simulink model "qdr_5_5"  (Simulink 7.9)
settings: Solver=ode45  StartTime=0.0  StopTime=10.0  RelTol=1e-3
libraries: xbsIndex_r4 x44, xps_library x2, casper_library_delays x2, casper_library_misc x1
settings Model: Creator=tfiliba  LastModifiedBy=tfiliba

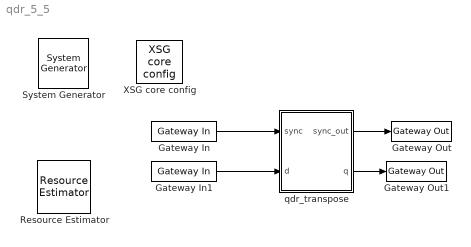
== system qdr_5_5 ==
  " System Generator" : xbsIndex_r4/ System Generator  Tag=genX  xilinxfamily=virtex5  part=xc5vsx95t  speed=-1  package=ff1136  synthesis_tool=XST  clock_wrapper=Clock Enables  directory=./netlist  proj_type=Project Navigator  Synth_file=XST Defaults  Impl_file=ISE Defaults  testbench=off  simulink_period=1  sysclk_period=10  dcm_input_clock_period=10  incr_netlist=off  trim_vbits=Everywhere in SubSystem  dbl_ovrd=According to Block Masks  core_generation=According to Block Masks  run_coregen=off  deprecated_control=off  eval_field=0  block_type=sysgen
  Gateway In : xbsIndex_r4/Gateway In  gui_display_data_type=Boolean  arith_type=Boolean  n_bits=16  bin_pt=14  preci_type=Single  exp_width=8  frac_width=24  quantization="Round  (unbiased: +/- Inf)"  overflow=Saturate  period=1  dbl_ovrd=off  timing_constraint=None  locs_specified=off  LOCs={}  UseAsADC=off  ADCChannel='1'  inherit_from_input=off  hdl_port=on  block_type=gatewayin
      settings: xl_area=[0 0 0 0 1 0 0]
  Gateway In1 : xbsIndex_r4/Gateway In  gui_display_data_type=Fixed-point  arith_type=Unsigned  n_bits=16  bin_pt=0  preci_type=Single  exp_width=8  frac_width=24  quantization="Round  (unbiased: +/- Inf)"  overflow=Saturate  period=1  dbl_ovrd=off  timing_constraint=None  locs_specified=off  LOCs={}  UseAsADC=off  ADCChannel='1'  inherit_from_input=off  hdl_port=on  block_type=gatewayin
      settings: xl_area=[0 0 0 0 16 0 0]
  Gateway Out : xbsIndex_r4/Gateway Out  inherit_from_input=off  hdl_port=on  timing_constraint=None  locs_specified=off  LOCs={}  UseAsDAC=off  DACChannel='1'  block_type=gatewayout
      settings: xl_area=[0 0 0 0 1 0 0]
  Gateway Out1 : xbsIndex_r4/Gateway Out  inherit_from_input=off  hdl_port=on  timing_constraint=None  locs_specified=off  LOCs={}  UseAsDAC=off  DACChannel='1'  block_type=gatewayout
      settings: xl_area=[0 0 0 0 36 0 0]
  Resource Estimator : xbsIndex_r4/Resource Estimator  Tag=resEstTag  Slices=0  FFs=0  BRAMs=0  LUTs=0  IOBs=0  EBMs=0  TBUFs=0  xl_use_estimator_area=off  est_options=Estimate  xl_estimator_area=[167 227 2 301 167 0 0]  block_type=resource_estimator
      settings: AttributesFormatString=Resource\nEstimator
  XSG core config : xps_library/XSG core config  Tag=xps:xsg  hw_sys=ROACH:sx95t  clk_src=arb_clk  ROACH_clk_src=arb_clk  ROACH2_clk_src=adc0_clk  clk_rate=200  sample_period=1  synthesis_tool=XST
  qdr_transpose : Subsystem  AncestorBlock=casper_library_reorder/qdr_transpose  mask{idepth=5, odepth=5, which_qdr=qdr1}
      mask prompts: idepth "Input blocksize (2^n)"; odepth "Output blocksize (2^n)"; which_qdr "QDR Chip"
      mask init:
      | new_map = tostring([[0:2^odepth-1]*2 [0:2^odepth-1]*2 + 1]);
      | set_param([gcb, '/reorder'], 'map', new_map);
      | set_param([gcb, '/qdr'], 'which_qdr', which_qdr);
      mask StyleString: edit,edit,popup(qdr0|qdr1)
  wires:
  Gateway In/1 -> qdr_transpose/1(sync)
  Gateway In1/1 -> qdr_transpose/2(d)
  qdr_transpose/1(sync_out) -> Gateway Out/1
  qdr_transpose/2(q) -> Gateway Out1/1

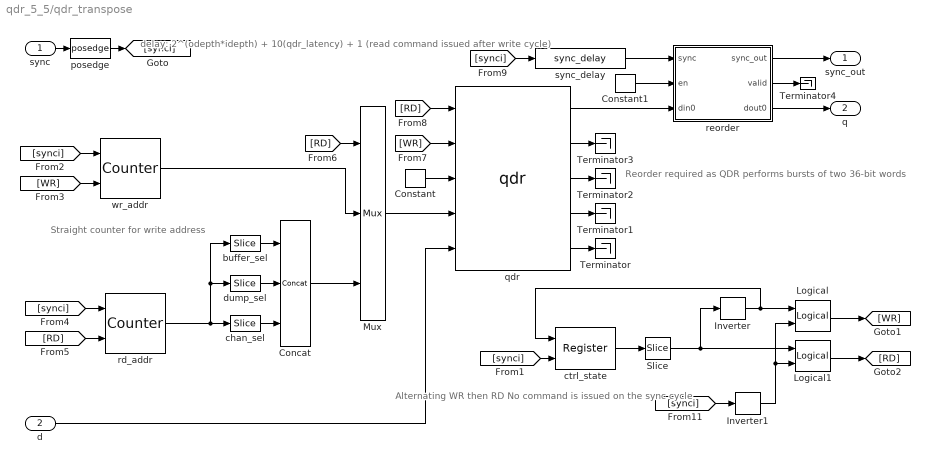
== system qdr_5_5/qdr_transpose ==
  note: delay: 2^(odepth*idepth) + 10(qdr_latency) + 1
      | (read command issued after write cycle)
  note: Reorder required as QDR performs
      | bursts of two 36-bit words
  note: Alternating WR then RD
      | No command is issued
      | on the sync cycle
  note: Straight counter for
      | write address
  sync : Inport
  d : Inport  Port=2
  Concat : xbsIndex_r4/Concat  num_inputs=3  dbl_ovrd=off  block_type=concat
      settings: block_version=10.1.3
  Constant : xbsIndex_r4/Constant  const=15  gui_display_data_type=Fixed-point  arith_type=Unsigned  n_bits=4  bin_pt=0  preci_type=Single  exp_width=8  frac_width=24  explicit_period=on  period=1  equ=P=C  opselect=C  inp2=PCIN>>17  opr=+  inp1=P  carry=CIN  dbl_ovrd=off  block_type=constant
  Constant1 : xbsIndex_r4/Constant  const=1  gui_display_data_type=Fixed-point  arith_type=Boolean  n_bits=4  bin_pt=0  preci_type=Single  exp_width=8  frac_width=24  explicit_period=on  period=1  equ=P=C  opselect=C  inp2=PCIN>>17  opr=+  inp1=P  carry=CIN  dbl_ovrd=off  block_type=constant
  Inverter : xbsIndex_r4/Inverter  en=off  latency=0  dbl_ovrd=off  block_type=inv
      settings: xl_area=[0 0 0 0 0 0 0]
  Inverter1 : xbsIndex_r4/Inverter  en=off  latency=0  dbl_ovrd=off  block_type=inv
      settings: xl_area=[0 0 0 0 0 0 0]
  Logical : xbsIndex_r4/Logical  logical_function=AND  inputs=2  en=off  latency=0  precision=Full  arith_type=Unsigned  n_bits=16  bin_pt=0  align_bp=on  dbl_ovrd=off  block_type=logical
      settings: xl_area=[1 0 0 1 0 0 0]
  Logical1 : xbsIndex_r4/Logical  logical_function=AND  inputs=2  en=off  latency=0  precision=Full  arith_type=Unsigned  n_bits=16  bin_pt=0  align_bp=on  dbl_ovrd=off  block_type=logical
      settings: xl_area=[1 0 0 1 0 0 0]
  Mux : xbsIndex_r4/Mux  inputs=2  en=off  latency=0  precision=Full  arith_type=Unsigned  n_bits=16  bin_pt=14  quantization=Truncate  overflow=Wrap  dbl_ovrd=off  block_type=mux
      settings: xl_area=[5 0 0 10 0 0 0]
  Slice : xbsIndex_r4/Slice  nbits=1  boolean_output=on  mode=Lower Bit Location + Width  bit1=0  base1=MSB of Input  bit0=0  base0=LSB of Input  dbl_ovrd=off  block_type=slice
      settings: infoedit="Extracts a given range of bits from each input sample and presents it at the output.  The output type is ordinarily unsigned with binary point at zero, but can be Boolean when the slice is one bit wide.<P><P>Hardware notes: In hardware this block costs nothing."  block_version=10.1.3
  Terminator{,1..4} (5 alike) : Terminator
  buffer_sel : xbsIndex_r4/Slice  nbits=1  boolean_output=off  mode=Upper Bit Location + Width  bit1=0  base1=MSB of Input  bit0=0  base0=LSB of Input  dbl_ovrd=off  block_type=slice
      settings: infoedit="Extracts a given range of bits from each input sample and presents it at the output.  The output type is ordinarily unsigned with binary point at zero, but can be Boolean when the slice is one bit wide.<P><P>Hardware notes: In hardware this block costs nothing."  block_version=10.1.3
  chan_sel : xbsIndex_r4/Slice  nbits=idepth - 1  boolean_output=off  mode=Lower Bit Location + Width  bit1=9-1  base1=MSB of Input  bit0=odepth  base0=LSB of Input  dbl_ovrd=off  block_type=slice
      settings: infoedit="Extracts a given range of bits from each input sample and presents it at the output.  The output type is ordinarily unsigned with binary point at zero, but can be Boolean when the slice is one bit wide.<P><P>Hardware notes: In hardware this block costs nothing."  block_version=10.1.3
  ctrl_state : xbsIndex_r4/Register  init=0  rst=on  en=off  dbl_ovrd=off  block_type=register
      settings: xl_area=[1 1 0 0 0 0 0]
  dump_sel : xbsIndex_r4/Slice  nbits=odepth  boolean_output=off  mode=Lower Bit Location + Width  bit1=0  base1=MSB of Input  bit0=0  base0=LSB of Input  dbl_ovrd=off  block_type=slice
      settings: infoedit="Extracts a given range of bits from each input sample and presents it at the output.  The output type is ordinarily unsigned with binary point at zero, but can be Boolean when the slice is one bit wide.<P><P>Hardware notes: In hardware this block costs nothing."  block_version=10.1.3
  posedge : casper_library_misc/posedge  Tag=Rising Edge Detector
      link override Delay: xl_area=[1 1 0 0 0 0 0]
      link override Inverter: xl_area=[0 0 0 0 0 0 0]
      link override Logical: xl_area=[1 0 0 1 0 0 0]
  qdr : xps_library/qdr  Tag=xps:qdr  which_qdr=qdr1  qdr_awidth=odepth+idepth+1  use_sniffer=off
      link override convert_be: n_bits=4
      link override convert_data_in: n_bits=36
      link override convert_data_in1: n_bits=36
      link override extract_parity: bitexpr=b = {a[35],a[26],a[17],a[8],a[34:27],a[25:18],a[16:9],a[7:0]}  arith_type1=Unsigned  arith_type2=Unsigned  arith_type3=Unsigned  arith_type4=Unsigned
      link override insert_parity: bitexpr=b = {a[35],a[31:24],a[34],a[23:16],a[33],a[15:8],a[32],a[7:0]}  arith_type1=Unsigned  arith_type2=Unsigned  arith_type3=Unsigned  arith_type4=Unsigned
      link override qdr_12_15_qdr_transpose_qdr_data_out: n_bits=36
      link override qdr_5_5_qdr_transpose_qdr_data_out: n_bits=36
      link override qdr_latency: latency=10
      link override Delay1: xl_area=[1 1 0 0 0 0 0]
      link override Inverter2: xl_area=[0 0 0 0 0 0 0]
      link override Logical: xl_area=[1 0 0 1 0 0 0]
      link override Logical1: xl_area=[1 0 0 1 0 0 0]
      link override convert_ack: xl_area=[0 0 0 0 0 0 0]
      link override convert_address: xl_area=[0 0 0 0 0 0 0]
      link override convert_be: xl_area=[0 0 0 0 0 0 0]
      link override convert_cal_fail: xl_area=[0 0 0 0 0 0 0]
      link override convert_data_in: xl_area=[0 0 0 0 0 0 0]
      link override convert_data_in1: xl_area=[0 0 0 0 0 0 0]
      link override convert_rd_en: xl_area=[0 0 0 0 0 0 0]
      link override convert_ready: xl_area=[0 0 0 0 0 0 0]
      link override convert_wr_en: xl_area=[0 0 0 0 0 0 0]
      link override prev_rd: xl_area=[1 1 0 0 0 0 0]
      link override qdr_12_15_qdr_transpose_qdr_ack: xl_area=[0 0 0 0 1 0 0]
      link override qdr_12_15_qdr_transpose_qdr_address: xl_area=[0 0 0 0 32 0 0]
      link override qdr_12_15_qdr_transpose_qdr_be: xl_area=[0 0 0 0 4 0 0]
      link override qdr_12_15_qdr_transpose_qdr_cal_fail: xl_area=[0 0 0 0 1 0 0]
      link override qdr_12_15_qdr_transpose_qdr_data_in: xl_area=[0 0 0 0 36 0 0]
      link override qdr_12_15_qdr_transpose_qdr_data_out: xl_area=[0 0 0 0 36 0 0]
      link override qdr_12_15_qdr_transpose_qdr_phy_ready: xl_area=[0 0 0 0 1 0 0]
      link override qdr_12_15_qdr_transpose_qdr_rd_en: xl_area=[0 0 0 0 1 0 0]
      link override qdr_12_15_qdr_transpose_qdr_wr_en: xl_area=[0 0 0 0 1 0 0]
      link override qdr_5_5_qdr_transpose_qdr_ack: xl_area=[0 0 0 0 1 0 0]
      link override qdr_5_5_qdr_transpose_qdr_address: xl_area=[0 0 0 0 32 0 0]
      link override qdr_5_5_qdr_transpose_qdr_be: xl_area=[0 0 0 0 4 0 0]
      link override qdr_5_5_qdr_transpose_qdr_cal_fail: xl_area=[0 0 0 0 1 0 0]
      link override qdr_5_5_qdr_transpose_qdr_data_in: xl_area=[0 0 0 0 36 0 0]
      link override qdr_5_5_qdr_transpose_qdr_data_out: xl_area=[0 0 0 0 36 0 0]
      link override qdr_5_5_qdr_transpose_qdr_phy_ready: xl_area=[0 0 0 0 1 0 0]
      link override qdr_5_5_qdr_transpose_qdr_rd_en: xl_area=[0 0 0 0 1 0 0]
      link override qdr_5_5_qdr_transpose_qdr_wr_en: xl_area=[0 0 0 0 1 0 0]
      link override qdr_latency: xl_area=[1 1 0 1 0 0 0]
  rd_addr : xbsIndex_r4/Counter  cnt_type=Free Running  cnt_to=Inf  operation=Up  start_count=2^(odepth + idepth - 1)  cnt_by_val=1  arith_type=Unsigned  n_bits=(idepth + odepth + 1) - 1  bin_pt=0  load_pin=off  rst=on  en=on  explicit_period=on  period=1  dbl_ovrd=off  use_behavioral_HDL=off  implementation=Fabric  use_rpm=off  block_type=counter
      settings: xl_area=[6 10 0 10 0 0 0]
  reorder : Subsystem  AncestorBlock=casper_library_reorder/reorder  mask(reorder){map=[0                                      2                                      4                                      6                                      8                                     10                                     12                                     14                                     16                                     18                                     20                                     22                                     24                                     26                                     28                                     30                                     32                                     34                                     36                                     38                                     40                                     42                                     44                                     46                                     48                                     50                                     52                                     54                                     56                                     58                                     60                                     62                                      1                                      3                                      5                                      7                                      9                                     11                                     13                                     15                                     17                                     19                                     21                                     23                                     25                                     27                                     29                                     31                                     33                                     35                                     37                                     39                                     41                                     43                                     45                                     47                                     49                                     51                                     53                                     55                                     57                                     59                                     61                                     63], n_inputs=1, bram_latency=2, map_latency=3, double_buffer=0, bram_map=off}
      mask prompts: map "Output Order:"; n_inputs "Number of inputs"; bram_latency "BRAM Latency"; map_latency "Map Latency"; double_buffer "Double Buffer"; bram_map "Use BlockRAM for Map"
      mask init:
      | reorder_init(gcb, ...
      |     'map', map, ...
      |     'n_inputs', n_inputs, ...
      |     'bram_latency', bram_latency, ...
      |     'map_latency', map_latency, ...
      |     'double_buffer', double_buffer, ...
      |     'bram_map', bram_map);
      settings: AttributesFormatString=order=6
      mask Help: eval('xlWeb(''http://casper.berkeley.edu/wiki/Reorder'')')
  sync_delay : casper_library_delays/sync_delay  DelayLen=2^(idepth + odepth) + 10 + 1
      link override Counter: xl_area=[6 11 0 12 0 0 0]
      link override Logical: xl_area=[1 0 0 1 0 0 0]
      link override Mux: xl_area=[1 0 0 1 0 0 0]
      link override Relational: xl_area=[3 0 0 6 0 0 0]
      link override Relational1: xl_area=[3 0 0 6 0 0 0]
  wr_addr : xbsIndex_r4/Counter  cnt_type=Free Running  cnt_to=Inf  operation=Up  start_count=0  cnt_by_val=1  arith_type=Unsigned  n_bits=(idepth + odepth + 1) - 1  bin_pt=0  load_pin=off  rst=on  en=on  explicit_period=on  period=1  dbl_ovrd=off  use_behavioral_HDL=off  implementation=Fabric  use_rpm=off  block_type=counter
      settings: xl_area=[6 10 0 10 0 0 0]
  sync_out : Outport
  q : Outport  Port=2
  wires:
  ctrl_state/1 -> Slice/1
  sync/1 -> posedge/1
  [synci] -> ctrl_state/2
  [synci] -> wr_addr/1
  [WR] -> wr_addr/2
  [synci] -> rd_addr/1
  [RD] -> rd_addr/2
  Inverter/1 -> ctrl_state/1, Logical/1
  [RD] -> Mux/1
  wr_addr/1 -> Mux/2
  [RD] -> qdr/1
  [WR] -> qdr/2
  Constant/1 -> qdr/3
  Mux/1 -> qdr/4
  d/1 -> qdr/5
  qdr/5 -> Terminator/1
  qdr/4 -> Terminator1/1
  qdr/3 -> Terminator2/1
  qdr/2 -> Terminator3/1
  [synci] -> sync_delay/1
  Slice/1 -> Inverter/1, Logical1/1
  [synci] -> Inverter1/1
  posedge/1 -> [synci]
  Logical1/1 -> [RD]
  Inverter1/1 -> Logical/2, Logical1/2
  Logical/1 -> [WR]
  Concat/1 -> Mux/3
  buffer_sel/1 -> Concat/1
  rd_addr/1 -> chan_sel/1, buffer_sel/1, dump_sel/1
  dump_sel/1 -> Concat/2
  chan_sel/1 -> Concat/3
  sync_delay/1 -> reorder/1(sync)
  Constant1/1 -> reorder/2(en)
  qdr/1 -> reorder/3(din0)
  reorder/1(sync_out) -> sync_out/1
  reorder/2(valid) -> Terminator4/1
  reorder/3(dout0) -> q/1

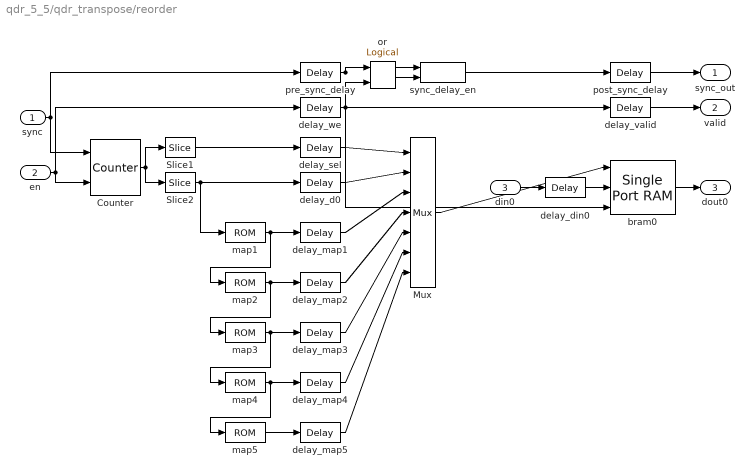
== system qdr_5_5/qdr_transpose/reorder ==
  sync : Inport
  en : Inport  Port=2
  din0 : Inport  Port=3
  Counter : xbsIndex_r4/Counter  cnt_type=Count Limited  cnt_to=383  operation=Up  start_count=0  cnt_by_val=1  arith_type=Unsigned  n_bits=9  bin_pt=0  load_pin=off  rst=on  en=on  explicit_period=on  period=1  dbl_ovrd=off  use_behavioral_HDL=off  implementation=Fabric  block_type=counter
      settings: xl_area=[8 9 0 12 0 0 0]
  Mux : xbsIndex_r4/Mux  inputs=6  en=off  latency=1  precision=Full  arith_type=Unsigned  n_bits=16  bin_pt=14  quantization=Truncate  overflow=Wrap  dbl_ovrd=off  block_type=mux
      settings: xl_area=[12 6 0 24 0 0 0]
  Slice1 : xbsIndex_r4/Slice  nbits=3  boolean_output=off  mode=Upper Bit Location + Width  bit1=0  base1=MSB of Input  bit0=0  base0=LSB of Input  dbl_ovrd=off  block_type=slice
  Slice2 : xbsIndex_r4/Slice  nbits=6  boolean_output=off  mode=Lower Bit Location + Width  bit1=0  base1=MSB of Input  bit0=0  base0=LSB of Input  dbl_ovrd=off  block_type=slice
  bram0 : xbsIndex_r4/Single Port RAM  depth=64  initVector=sin(pi*(0:15)/16)  distributed_mem=Block RAM  write_mode=Read Before Write  rst=off  init_reg=0  en=off  latency=2  dbl_ovrd=off  optimize=Area  use_rpm=on  block_type=spram
      settings: xl_area=[0 36 2 0 0 0 0]
  delay_d0 : xbsIndex_r4/Delay  rst=off  infoeditControl=Selection of Reset will increase slice count due to use of real FFs and instead of SRLs  en=off  latency=15  dbl_ovrd=off  reg_retiming=off  block_type=delay
      settings: xl_area=[3 6 0 6 0 0 0]
  delay_din0 : xbsIndex_r4/Delay  rst=off  infoeditControl=Selection of Reset will increase slice count due to use of real FFs and instead of SRLs  en=off  latency=16  dbl_ovrd=off  reg_retiming=off  block_type=delay
      settings: xl_area=[18 36 0 36 0 0 0]
  delay_map1 : xbsIndex_r4/Delay  rst=off  infoeditControl=Selection of Reset will increase slice count due to use of real FFs and instead of SRLs  en=off  latency=4*map_latency  dbl_ovrd=off  reg_retiming=off  block_type=delay
      settings: xl_area=[3 6 0 6 0 0 0]
  delay_map2 : xbsIndex_r4/Delay  rst=off  infoeditControl=Selection of Reset will increase slice count due to use of real FFs and instead of SRLs  en=off  latency=3*map_latency  dbl_ovrd=off  reg_retiming=off  block_type=delay
      settings: xl_area=[3 6 0 6 0 0 0]
  delay_map3 : xbsIndex_r4/Delay  rst=off  infoeditControl=Selection of Reset will increase slice count due to use of real FFs and instead of SRLs  en=off  latency=2*map_latency  dbl_ovrd=off  reg_retiming=off  block_type=delay
      settings: xl_area=[3 6 0 6 0 0 0]
  delay_map4 : xbsIndex_r4/Delay  rst=off  infoeditControl=Selection of Reset will increase slice count due to use of real FFs and instead of SRLs  en=off  latency=1*map_latency  dbl_ovrd=off  reg_retiming=off  block_type=delay
      settings: xl_area=[3 6 0 6 0 0 0]
  delay_map5 : xbsIndex_r4/Delay  rst=off  infoeditControl=Selection of Reset will increase slice count due to use of real FFs and instead of SRLs  en=off  latency=0*map_latency  dbl_ovrd=off  reg_retiming=off  block_type=delay
      settings: xl_area=[0 0 0 0 0 0 0]
  delay_sel : xbsIndex_r4/Delay  rst=off  infoeditControl=Selection of Reset will increase slice count due to use of real FFs and instead of SRLs  en=off  latency=15  dbl_ovrd=off  reg_retiming=off  block_type=delay
      settings: xl_area=[2 3 0 3 0 0 0]
  delay_valid : xbsIndex_r4/Delay  rst=off  infoeditControl=Selection of Reset will increase slice count due to use of real FFs and instead of SRLs  en=off  latency=2  dbl_ovrd=off  reg_retiming=off  block_type=delay
      settings: xl_area=[1 1 0 1 0 0 0]
  delay_we : xbsIndex_r4/Delay  rst=off  infoeditControl=Selection of Reset will increase slice count due to use of real FFs and instead of SRLs  en=off  latency=16  dbl_ovrd=off  reg_retiming=off  block_type=delay
      settings: xl_area=[1 1 0 1 0 0 0]
  map{1..5} (5 alike) : xbsIndex_r4/ROM  depth=64  initVector=map  distributed_mem=Distributed memory  rst=off  init_reg=0  en=off  latency=3  gui_display_data_type=Fixed-point  arith_type=Unsigned  n_bits=6  bin_pt=0  preci_type=Single  exp_width=8  frac_width=24  dbl_ovrd=off  optimize=Area  use_rpm=on  block_type=sprom
      settings: xl_area=[11 12 0 22 0 0 0]
  or : xbsIndex_r4/Logical  logical_function=OR  inputs=2  en=off  latency=0  precision=Full  arith_type=Unsigned  n_bits=16  bin_pt=0  align_bp=on  dbl_ovrd=off  block_type=logical
      settings: xl_area=[1 0 0 1 0 0 0]
  post_sync_delay : xbsIndex_r4/Delay  rst=off  infoeditControl=Selection of Reset will increase slice count due to use of real FFs and instead of SRLs  en=off  latency=2  dbl_ovrd=off  reg_retiming=off  block_type=delay
      settings: xl_area=[1 1 0 1 0 0 0]
  pre_sync_delay : xbsIndex_r4/Delay  rst=off  infoeditControl=Selection of Reset will increase slice count due to use of real FFs and instead of SRLs  en=off  latency=16  dbl_ovrd=off  reg_retiming=off  block_type=delay
      settings: xl_area=[1 1 0 1 0 0 0]
  sync_delay_en : casper_library_delays/sync_delay_en  DelayLen=64
      link override Counter: xl_area=[4 7 0 8 0 0 0]
      link override Logical: xl_area=[1 0 0 1 0 0 0]
      link override Logical1: xl_area=[1 0 0 1 0 0 0]
      link override Mux: xl_area=[1 0 0 1 0 0 0]
      link override Relational: xl_area=[2 0 0 4 0 0 0]
      link override Relational1: xl_area=[2 0 0 4 0 0 0]
  sync_out : Outport
  valid : Outport  Port=2
  dout0 : Outport  Port=3
  wires:
  en/1 -> delay_we/1, Counter/2
  delay_we/1 -> delay_valid/1, or/2, bram0/3
  delay_valid/1 -> valid/1
  sync/1 -> pre_sync_delay/1, Counter/1
  pre_sync_delay/1 -> or/1, sync_delay_en/1
  or/1 -> sync_delay_en/2
  sync_delay_en/1 -> post_sync_delay/1
  post_sync_delay/1 -> sync_out/1
  Counter/1 -> Slice1/1, Slice2/1
  Slice1/1 -> delay_sel/1
  delay_sel/1 -> Mux/1
  Slice2/1 -> delay_d0/1, map1/1
  delay_d0/1 -> Mux/2
  Mux/1 -> bram0/1
  din0/1 -> delay_din0/1
  delay_din0/1 -> bram0/2
  bram0/1 -> dout0/1
  map1/1 -> delay_map1/1, map2/1
  delay_map1/1 -> Mux/3
  map2/1 -> delay_map2/1, map3/1
  delay_map2/1 -> Mux/4
  map3/1 -> delay_map3/1, map4/1
  delay_map3/1 -> Mux/5
  map4/1 -> delay_map4/1, map5/1
  delay_map4/1 -> Mux/6
  map5/1 -> delay_map5/1
  delay_map5/1 -> Mux/7
